simulink library "Driveshaft_Assembly_3D"  (R2026a)
settings: Solver=VariableStepAuto
undefined symbols (not defined in the file): Driveshaft, Housing, Right, Shaft, Visual
libraries: sm_lib x10, Suspension_Utilities x2, Driveshaft_Shaft x1
Description:
  | Component of Simscape Vehicle Templates Library
  | 
  | Copyright 2018-2026 The MathWorks, Inc.
settings Model: Creator=smiller  LastModifiedBy=smiller

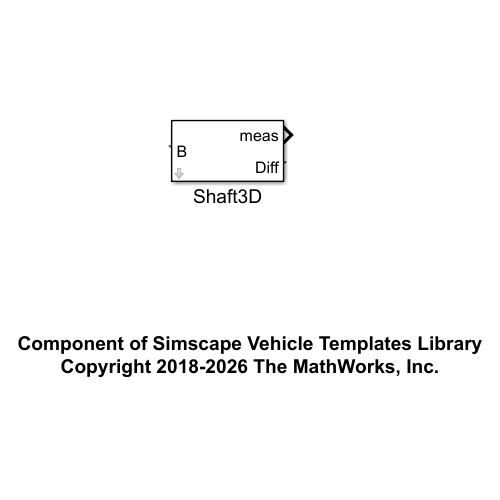
[thumbnail: Simulink's stored preview of the top-level diagram]
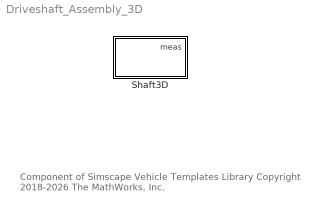
== system Driveshaft_Assembly_3D ==
  note: Component of Simscape Vehicle Templates Library
      | Copyright 2018-2026 The MathWorks, Inc.
  Shaft3D : Subsystem  VariantControl=Shaft3D  mask(Driveshaft Assembly (3D)){popup_leftRight=Right, Driveshaft=Driveshaft, clr_drv_sha_hp=Visual.hp.clr, opc_drv_sha_hp=Visual.hp.opc, rad_drv_sha_hp=Visual.hp.rad, clr_drv_sha_jnt=Visual.DriveshaftCVs.clr, opc_drv_sha_jnt=Visual.part.opc, rad_drv_sha_jnt=Visual.DriveshaftCVs.rad, clr_drv_sha_drvsh=Visual.Driveshaft.clr, opc_drv_sha_drvsh=Visual.part.opc, rad_drv_sha_drvsh=Visual.Driveshaft.rad}
      mask prompts: popup_leftRight "Left/Right"; Driveshaft "Driveshaft Parameters"
      mask help: Models a driveshaft assembly with CV joints and a shaft. The joints can be configured to permit plunge at the inboard or outboard joint. The shaft can be rigid or flexible.
      mask TypeOptions popup_leftRight: AxleInboard/popup_leftRight | Shaft/popup_leftRight
      mask TypeOptions clr_drv_sha_hp:
      | Vis HP
      | Transaxle/GraphicDiffuseColor
      mask TypeOptions opc_drv_sha_hp:
      | Vis HP
      | Transaxle/GraphicOpacity
      mask TypeOptions rad_drv_sha_hp:
      | Vis HP
      | Transaxle/SphereRadius
      mask TypeOptions clr_drv_sha_jnt:
      | Vis CV Joint
      | Inboard/GraphicDiffuseColor | Vis CV Joint
      | Outboard/GraphicDiffuseColor
      mask TypeOptions opc_drv_sha_jnt:
      | Vis CV Joint
      | Inboard/GraphicOpacity | Vis CV Joint
      | Outboard/GraphicOpacity
      mask TypeOptions rad_drv_sha_jnt:
      | Vis CV Joint
      | Inboard/SphereRadius | Vis CV Joint
      | Outboard/SphereRadius
      mask TypeOptions clr_drv_sha_drvsh: Shaft/clr_shaft
      mask TypeOptions opc_drv_sha_drvsh: Shaft/opc_shaft
      mask TypeOptions rad_drv_sha_drvsh: Shaft/rad_shaft
      mask DialogControl cont_vis_drv_sha Prompt: Visualization
      mask DialogControl text_vis_drv_sha_clr Prompt: Color [RGB]
      mask DialogControl text_vis_drv_sha_opc Prompt: Opac. (0-1)
      mask DialogControl text_vis_drv_sha_rad Prompt: Radius (m)
      mask DialogControl text_vis_drv_sha_hp Prompt: Hardpoints
      mask DialogControl text_vis_drv_sha_joints Prompt: Joints
      mask DialogControl text_vis_drv_sha_drvsh Prompt: Driveshaft

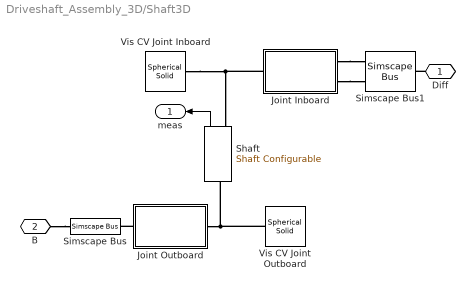
== system Driveshaft_Assembly_3D/Shaft3D ==
  Joint Inboard : Subsystem  Variant=on  VariantControlMode=label  VariantControl=Variant1  LabelModeActiveChoice=CV  mask{VariantLabel=Driveshaft.JointInboard.class.Value}
      mask prompts: VariantLabel "Variant Label"
      mask init:
      | curblk = gcb;
      | 
      | % Set variant for this block 
      | set_param(curblk,'LabelModeActiveChoice',VariantLabel);
      settings: AttributesFormatString=%<ActiveVariant>
      mask Display: disp(' ');
  Joint Outboard : Subsystem  Variant=on  VariantControlMode=label  VariantControl=Variant1  LabelModeActiveChoice=CV  mask{VariantLabel=Driveshaft.JointOutboard.class.Value}
      mask prompts: VariantLabel "Variant Label"
      mask init:
      | curblk = gcb;
      | 
      | % Set variant for this block 
      | set_param(curblk,'LabelModeActiveChoice',VariantLabel);
      settings: AttributesFormatString=%<ActiveVariant>
      mask Display: disp(' ');
  Shaft : Driveshaft_Shaft/Shaft Configurable  VariantControl=Variant1  LabelModeActiveChoice=Rigid  popup_leftRight=Right  Shaft=Driveshaft.Shaft  VariantLabel=Driveshaft.Shaft.class.Value  clr_shaft=clr_drv_sha_drvsh  opc_shaft=opc_drv_sha_drvsh  rad_shaft=rad_drv_sha_drvsh
      settings: AttributesFormatString=%<ActiveVariant>
  Simscape Bus : SimscapeBus  HierarchyStrings=AxleIn
  Simscape Bus1 : SimscapeBus  HierarchyStrings=Shaft;Housing
  Vis CV Joint Inboard : sm_lib/Body Elements/Spherical Solid  SphereRadius=rad_drv_sha_jnt  SphereRadiusUnits=m  ExportEntireGeometry=off  InertiaType=CalculateFromGeometry  BasedOnType=Density  Density=0  DensityUnits=kg/m^3  Mass=1  MassUnits=kg  CenterOfMass=[0 0 0]  CenterOfMassUnits=m  MomentsOfInertia=[1 1 1]  MomentsOfInertiaUnits=kg*m^2  ProductsOfInertia=[0 0 0]  ProductsOfInertiaUnits=kg*m^2  GraphicType=FromGeometry  MarkerShape=Sphere  MarkerSize=10  GraphicVisPropType=SimpleVisualProperties  GraphicDiffuseColor=clr_drv_sha_jnt  GraphicOpacity=opc_drv_sha_jnt  GraphicSpecularColor=[0.5 0.5 0.5 1.0]  GraphicAmbientColor=[0.15 0.15 0.15 1.0]  GraphicEmissiveColor=[0.0 0.0 0.0 1.0]  GraphicShininess=75  DoExposeReferenceFrame=on  SerializedFrames=<Frames/>
  Vis CV Joint Outboard : sm_lib/Body Elements/Spherical Solid  SphereRadius=rad_drv_sha_jnt  SphereRadiusUnits=m  ExportEntireGeometry=off  InertiaType=CalculateFromGeometry  BasedOnType=Density  Density=0  DensityUnits=kg/m^3  Mass=1  MassUnits=kg  CenterOfMass=[0 0 0]  CenterOfMassUnits=m  MomentsOfInertia=[1 1 1]  MomentsOfInertiaUnits=kg*m^2  ProductsOfInertia=[0 0 0]  ProductsOfInertiaUnits=kg*m^2  GraphicType=FromGeometry  MarkerShape=Sphere  MarkerSize=10  GraphicVisPropType=SimpleVisualProperties  GraphicDiffuseColor=clr_drv_sha_jnt  GraphicOpacity=opc_drv_sha_jnt  GraphicSpecularColor=[0.5 0.5 0.5 1.0]  GraphicAmbientColor=[0.15 0.15 0.15 1.0]  GraphicEmissiveColor=[0.0 0.0 0.0 1.0]  GraphicShininess=75  DoExposeReferenceFrame=on  SerializedFrames=<Frames/>
  Diff : PMIOPort  Side=Right
  B : PMIOPort  Port=2  Side=Left
  meas : Outport  VectorParamsAs1DForOutWhenUnconnected=off
  wires:
  Shaft/1 -> meas/1
  connections:
  Joint Outboard/LConn1 -- Simscape Bus/LConn1
  Joint Outboard/RConn1 -- Shaft/LConn1 -- Vis CV Joint Outboard/RConn1
  Joint Inboard/RConn2 -- Simscape Bus1/LConn2
  Joint Inboard/RConn1 -- Simscape Bus1/LConn1
  Joint Inboard/LConn1 -- Shaft/RConn1 -- Vis CV Joint Inboard/RConn1
  Diff/RConn1 -- Simscape Bus1/RConn1
  B/RConn1 -- Simscape Bus/RConn1

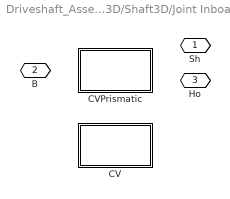
== system Driveshaft_Assembly_3D/Shaft3D/Joint Inboard ==
  CV : Subsystem  VariantControl=CV
  CVPrismatic : Subsystem  VariantControl=CVPrismatic
  " Sh" : PMIOPort  Side=Right
  " B" : PMIOPort  Port=2  Side=Left
  " Ho" : PMIOPort  Port=3  Side=Right

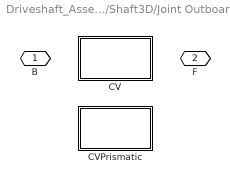
== system Driveshaft_Assembly_3D/Shaft3D/Joint Outboard ==
  CV : Subsystem  VariantControl=CV
  CVPrismatic : Subsystem  VariantControl=CVPrismatic
  " B" : PMIOPort  Side=Left
  " F" : PMIOPort  Port=2  Side=Right

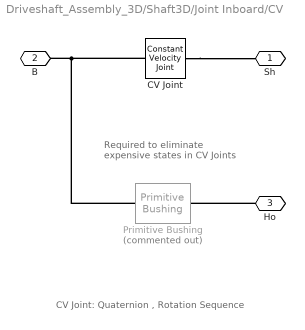
== system Driveshaft_Assembly_3D/Shaft3D/Joint Inboard/CV ==
  note: CV Joint: Quaternion , Rotation Sequence
  note: Required to eliminate
      | expensive states
      | in CV Joints
  CV Joint : sm_lib/Joints/Constant Velocity Joint  JointMode=Normal  CompositeWrenchDir=FollowerOnBase  CompositeWrenchFrame=BaseFrame  SenseConstraintForce=off  SenseConstraintTorque=off  SenseTotalForce=off  SenseTotalTorque=off  InternalState=RotationSequence  PositionTargetSpecify=off  PositionTargetPriority=High  PositionTargetSpecificationMethod=BendAngleOnly  PositionTargetBendAngleValue=0.0  PositionTargetBendAngleValueUnits=deg  PositionTargetAzimuthValue=0.0  PositionTargetAzimuthValueUnits=deg  VelocityTargetSpecify=off  VelocityTargetPriority=High  VelocityTargetSpecificationMethod=BendAngleOnly  VelocityTargetBendAngleValue=0.0  VelocityTargetBendAngleValueUnits=deg/s  VelocityTargetAzimuthValue=0.0  VelocityTargetAzimuthValueUnits=deg/s  SenseBendAnglePosition=off  SenseBendAngleVelocity=off  SenseBendAngleAcceleration=off  SenseAzimuthPosition=off  SenseAzimuthVelocity=off  SenseAzimuthAcceleration=off
      settings: AttributesFormatString=%<InternalState>
  Primitive Bushing : Suspension_Utilities/Primitive Bushing  Commented=on  SystemSampleTime=-1  VariantActivationTime=update diagram  EmptyChoice=off  PassThrough=off  PassThroughVariantControl=(default)  EmptyChoiceVariantControl=(default)  AllowFlexibleInterface=on  Latency=0  AutoFrameSizeCalculation=off
  Sh : PMIOPort  Side=Right
  B : PMIOPort  Port=2  Side=Left
  Ho : PMIOPort  Port=3  Side=Right
  connections:
  Ho/RConn1 -- Primitive Bushing/LConn1
  CV Joint/LConn1 -- B/RConn1 -- Primitive Bushing/RConn1
  CV Joint/RConn1 -- Sh/RConn1

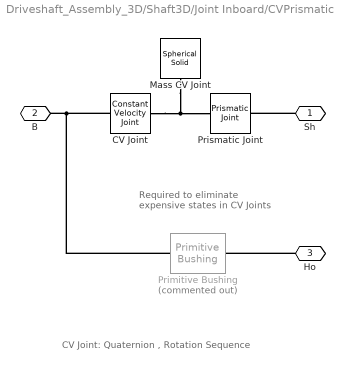
== system Driveshaft_Assembly_3D/Shaft3D/Joint Inboard/CVPrismatic ==
  note: Required to eliminate
      | expensive states
      | in CV Joints
  note: CV Joint: Quaternion , Rotation Sequence
  CV Joint : sm_lib/Joints/Constant Velocity Joint  JointMode=Normal  CompositeWrenchDir=FollowerOnBase  CompositeWrenchFrame=BaseFrame  SenseConstraintForce=off  SenseConstraintTorque=off  SenseTotalForce=off  SenseTotalTorque=off  InternalState=RotationSequence  PositionTargetSpecify=off  PositionTargetPriority=High  PositionTargetSpecificationMethod=BendAngleOnly  PositionTargetBendAngleValue=0.0  PositionTargetBendAngleValueUnits=deg  PositionTargetAzimuthValue=0.0  PositionTargetAzimuthValueUnits=deg  VelocityTargetSpecify=off  VelocityTargetPriority=High  VelocityTargetSpecificationMethod=BendAngleOnly  VelocityTargetBendAngleValue=0.0  VelocityTargetBendAngleValueUnits=deg/s  VelocityTargetAzimuthValue=0.0  VelocityTargetAzimuthValueUnits=deg/s  SenseBendAnglePosition=off  SenseBendAngleVelocity=off  SenseBendAngleAcceleration=off  SenseAzimuthPosition=off  SenseAzimuthVelocity=off  SenseAzimuthAcceleration=off
      settings: AttributesFormatString=%<InternalState>
  Mass CV Joint : sm_lib/Body Elements/Spherical Solid  SphereRadius=5e-3  SphereRadiusUnits=m  ExportEntireGeometry=off  InertiaType=CalculateFromGeometry  BasedOnType=Density  Density=1000  DensityUnits=kg/m^3  Mass=1  MassUnits=kg  CenterOfMass=[0 0 0]  CenterOfMassUnits=m  MomentsOfInertia=[1 1 1]  MomentsOfInertiaUnits=kg*m^2  ProductsOfInertia=[0 0 0]  ProductsOfInertiaUnits=kg*m^2  GraphicType=FromGeometry  MarkerShape=Sphere  MarkerSize=10  GraphicVisPropType=SimpleVisualProperties  GraphicDiffuseColor=[0.5 0.5 0.5]  GraphicOpacity=1  GraphicSpecularColor=[0.5 0.5 0.5 1.0]  GraphicAmbientColor=[0.15 0.15 0.15 1.0]  GraphicEmissiveColor=[0.0 0.0 0.0 1.0]  GraphicShininess=75  DoExposeReferenceFrame=on  SerializedFrames=<Frames/>
  Primitive Bushing : Suspension_Utilities/Primitive Bushing  Commented=on  SystemSampleTime=-1  VariantActivationTime=update diagram  EmptyChoice=off  PassThrough=off  PassThroughVariantControl=(default)  EmptyChoiceVariantControl=(default)  AllowFlexibleInterface=on  Latency=0  AutoFrameSizeCalculation=off
  Prismatic Joint : sm_lib/Joints/Prismatic Joint  JointMode=Normal  CompositeWrenchDir=FollowerOnBase  CompositeWrenchFrame=BaseFrame  SenseConstraintForce=off  SenseConstraintTorque=off  SenseTotalForce=off  SenseTotalTorque=off  PositionTargetSpecify=off  PositionTargetPriority=High  PositionTargetValue=0  PositionTargetValueUnits=m  VelocityTargetSpecify=off  VelocityTargetPriority=High  VelocityTargetValue=0  VelocityTargetValueUnits=m/s  EquilibriumPosition=0  EquilibriumPositionUnits=m  SpringStiffness=0  SpringStiffnessUnits=N/m  DampingCoefficient=0  DampingCoefficientUnits=N/(m/s)  LowerLimitSpecify=off  LowerLimitBound=-1  LowerLimitBoundUnits=m  LowerLimitStiffness=1e6  LowerLimitStiffnessUnits=N/m  LowerLimitDamping=1e3  LowerLimitDampingUnits=N/(m/s)  LowerLimitTransitionRegionWidth=1e-4  LowerLimitTransitionRegionWidthUnits=m  UpperLimitSpecify=off  UpperLimitBound=1  UpperLimitBoundUnits=m  UpperLimitStiffness=1e6  UpperLimitStiffnessUnits=N/m  UpperLimitDamping=1e3  UpperLimitDampingUnits=N/(m/s)  UpperLimitTransitionRegionWidth=1e-4  UpperLimitTransitionRegionWidthUnits=m  TorqueActuationMode=NoTorque  MotionActuationMode=ComputedMotion  SensePosition=off  SenseVelocity=off  SenseAcceleration=off  SenseTorqueForce=off  SenseLowerLimitTorqueForce=off  SenseUpperLimitTorqueForce=off
  Sh : PMIOPort  Side=Right
  B : PMIOPort  Port=2  Side=Left
  Ho : PMIOPort  Port=3  Side=Right
  connections:
  Sh/RConn1 -- Prismatic Joint/RConn1
  CV Joint/RConn1 -- Prismatic Joint/LConn1 -- Mass CV Joint/RConn1
  CV Joint/LConn1 -- Primitive Bushing/RConn1 -- B/RConn1
  Ho/RConn1 -- Primitive Bushing/LConn1

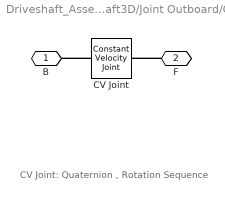
== system Driveshaft_Assembly_3D/Shaft3D/Joint Outboard/CV ==
  note: CV Joint: Quaternion , Rotation Sequence
  CV Joint : sm_lib/Joints/Constant Velocity Joint  JointMode=Normal  CompositeWrenchDir=FollowerOnBase  CompositeWrenchFrame=BaseFrame  SenseConstraintForce=off  SenseConstraintTorque=off  SenseTotalForce=off  SenseTotalTorque=off  InternalState=RotationSequence  PositionTargetSpecify=off  PositionTargetPriority=High  PositionTargetSpecificationMethod=BendAngleOnly  PositionTargetBendAngleValue=0.0  PositionTargetBendAngleValueUnits=deg  PositionTargetAzimuthValue=0.0  PositionTargetAzimuthValueUnits=deg  VelocityTargetSpecify=off  VelocityTargetPriority=High  VelocityTargetSpecificationMethod=BendAngleOnly  VelocityTargetBendAngleValue=0.0  VelocityTargetBendAngleValueUnits=deg/s  VelocityTargetAzimuthValue=0.0  VelocityTargetAzimuthValueUnits=deg/s  SenseBendAnglePosition=off  SenseBendAngleVelocity=off  SenseBendAngleAcceleration=off  SenseAzimuthPosition=off  SenseAzimuthVelocity=off  SenseAzimuthAcceleration=off
      settings: AttributesFormatString=%<InternalState>
  B : PMIOPort  Side=Left
  F : PMIOPort  Port=2  Side=Right
  connections:
  CV Joint/LConn1 -- B/RConn1
  F/RConn1 -- CV Joint/RConn1

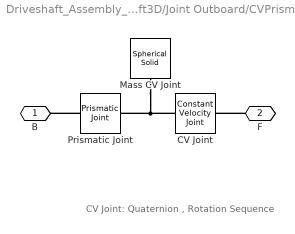
== system Driveshaft_Assembly_3D/Shaft3D/Joint Outboard/CVPrismatic ==
  note: CV Joint: Quaternion , Rotation Sequence
  CV Joint : sm_lib/Joints/Constant Velocity Joint  JointMode=Normal  CompositeWrenchDir=FollowerOnBase  CompositeWrenchFrame=BaseFrame  SenseConstraintForce=off  SenseConstraintTorque=off  SenseTotalForce=off  SenseTotalTorque=off  InternalState=RotationSequence  PositionTargetSpecify=off  PositionTargetPriority=High  PositionTargetSpecificationMethod=BendAngleOnly  PositionTargetBendAngleValue=0.0  PositionTargetBendAngleValueUnits=deg  PositionTargetAzimuthValue=0.0  PositionTargetAzimuthValueUnits=deg  VelocityTargetSpecify=off  VelocityTargetPriority=High  VelocityTargetSpecificationMethod=BendAngleOnly  VelocityTargetBendAngleValue=0.0  VelocityTargetBendAngleValueUnits=deg/s  VelocityTargetAzimuthValue=0.0  VelocityTargetAzimuthValueUnits=deg/s  SenseBendAnglePosition=off  SenseBendAngleVelocity=off  SenseBendAngleAcceleration=off  SenseAzimuthPosition=off  SenseAzimuthVelocity=off  SenseAzimuthAcceleration=off
      settings: AttributesFormatString=%<InternalState>
  Mass CV Joint : sm_lib/Body Elements/Spherical Solid  SphereRadius=5e-3  SphereRadiusUnits=m  ExportEntireGeometry=off  InertiaType=CalculateFromGeometry  BasedOnType=Density  Density=1*1000  DensityUnits=kg/m^3  Mass=1  MassUnits=kg  CenterOfMass=[0 0 0]  CenterOfMassUnits=m  MomentsOfInertia=[1 1 1]  MomentsOfInertiaUnits=kg*m^2  ProductsOfInertia=[0 0 0]  ProductsOfInertiaUnits=kg*m^2  GraphicType=FromGeometry  MarkerShape=Sphere  MarkerSize=10  GraphicVisPropType=SimpleVisualProperties  GraphicDiffuseColor=[0.5 0.5 0.5]  GraphicOpacity=1  GraphicSpecularColor=[0.5 0.5 0.5 1.0]  GraphicAmbientColor=[0.15 0.15 0.15 1.0]  GraphicEmissiveColor=[0.0 0.0 0.0 1.0]  GraphicShininess=75  DoExposeReferenceFrame=on  SerializedFrames=<Frames/>
  Prismatic Joint : sm_lib/Joints/Prismatic Joint  JointMode=Normal  CompositeWrenchDir=FollowerOnBase  CompositeWrenchFrame=BaseFrame  SenseConstraintForce=off  SenseConstraintTorque=off  SenseTotalForce=off  SenseTotalTorque=off  PositionTargetSpecify=off  PositionTargetPriority=High  PositionTargetValue=0  PositionTargetValueUnits=m  VelocityTargetSpecify=off  VelocityTargetPriority=High  VelocityTargetValue=0  VelocityTargetValueUnits=m/s  EquilibriumPosition=0  EquilibriumPositionUnits=m  SpringStiffness=0  SpringStiffnessUnits=N/m  DampingCoefficient=0  DampingCoefficientUnits=N/(m/s)  LowerLimitSpecify=off  LowerLimitBound=-1  LowerLimitBoundUnits=m  LowerLimitStiffness=1e6  LowerLimitStiffnessUnits=N/m  LowerLimitDamping=1e3  LowerLimitDampingUnits=N/(m/s)  LowerLimitTransitionRegionWidth=1e-4  LowerLimitTransitionRegionWidthUnits=m  UpperLimitSpecify=off  UpperLimitBound=1  UpperLimitBoundUnits=m  UpperLimitStiffness=1e6  UpperLimitStiffnessUnits=N/m  UpperLimitDamping=1e3  UpperLimitDampingUnits=N/(m/s)  UpperLimitTransitionRegionWidth=1e-4  UpperLimitTransitionRegionWidthUnits=m  TorqueActuationMode=NoTorque  MotionActuationMode=ComputedMotion  SensePosition=off  SenseVelocity=off  SenseAcceleration=off  SenseTorqueForce=off  SenseLowerLimitTorqueForce=off  SenseUpperLimitTorqueForce=off
  B : PMIOPort  Side=Left
  F : PMIOPort  Port=2  Side=Right
  connections:
  Prismatic Joint/LConn1 -- B/RConn1
  F/RConn1 -- CV Joint/RConn1
  Mass CV Joint/RConn1 -- CV Joint/LConn1 -- Prismatic Joint/RConn1
